simulink model "simulering_ROV_DP_model2"  (R2020a)
settings: Solver=VariableStepAuto  StartTime=0.0  StopTime=t_sim  RelTol=1e-3
values from neighbouring files (symbols this model uses):
  B_aug = [b11 b12 b13 b14 b15 b16 ... (first row only)    [constants.m]
  B_psinv_aug = B_aug'/(B_aug*B_aug')    [constants.m]
  coriolis_effect = 1    [run_simulation.m]    (also in run_simulation_STA_controller.m; run_simulation_dp_model.m)
  d_11 = 250    [constants.m]    (also in constants_dp_model.m; constants_model_coriolis.m; constants_process_model.m)
  d_22 = 200    [constants.m]    (also in constants_dp_model.m; constants_model_coriolis.m; constants_process_model.m)
  d_33 = 175    [constants.m]    (also in constants_dp_model.m; constants_model_coriolis.m; constants_process_model.m)
  d_66 = 15    [constants.m]    (also in constants_process_model.m)
  d_n11 = 350    [constants.m]
  d_n22 = 350    [constants.m]
  d_n33 = 400    [constants.m]
  d_n66 = 75    [constants.m]
  Delta = 25    [plot_simulation_feedback.m]    (also in run_simulation.m; run_simulation_SM_controller.m; run_simulation_STA_controller.m; run_simulation_dp_model.m)
  g_z = 9.81    [run_simulation_FL_controller.m]    (also in run_simulation_PID_controller.m = 0.91; run_simulation_SM_controller.m = 0.91; run_simulation_STA_controller.m = 0.91; run_simulation_dp_model.m = 0.91)
  gamma1 = 50    [run_simulation_dp_model.m]    (also in tuning_dp_model.m = 5)
  gamma2 = 35    [run_simulation_dp_model.m]    (also in tuning_dp_model.m = 3.5)
  gamma_e1 = 0.05    [tuning_dp_model.m]
  gamma_e2 = 0.05    [tuning_dp_model.m]
  gamma_e3 = 0.05    [tuning_dp_model.m]
  k_d_psi = 2*m_44*zeta_d_psi*wn_psi-d_44    [run_simulation_PID_controller.m]    (also in run_simulation_SM_controller.m = 10; run_simulation_dp_model.m = 2*m_66*zeta_d_psi*wn_psi-d_66; run_simulation_feedback_linearizing.m = (2*1*k_p_psi*1-d33/(m_A33+m_RB33)); tuning_PID_controller.m = 2*m_66*zeta_d_psi*wn_psi-d_66)
  k_d_z = 30    [run_simulation_SM_controller.m]    (also in run_simulation_dp_model.m = 2*m_33*zeta_d_heave*wn_heave-d_33; tuning_FL_controller.m = 2*m_33*zeta_d_heave*wn_heave-d_33; tuning_SM_controller.m; tuning_dp_model.m = 2*m_33*zeta_d_heave*wn_heave-d_33)
  k_i_z = wn_heave/10*k_p_z    [run_simulation_PID_controller.m]    (also in run_simulation_dp_model.m = wn_heave/50*k_p_z; tuning_FL_controller.m = wn_heave/50*k_p_z; tuning_PID_controller.m = wn_heave/50*k_p_z; tuning_dp_model.m = wn_heave/50*k_p_z)
  k_p_psi = wn_psi^2-lambda*k_p_r    [run_simulation_FL_controller.m]    (also in run_simulation_PID_controller.m = wn_psi^2*m_44; run_simulation_dp_model.m = wn_psi^2*m_66; run_simulation_feedback_linearizing.m = tau_r_max/deg2rad(45); run_simulation_feedback_linearizing_second_try.m = wn_psi^2*m_44)
  k_p_u = m_11*pole_u-d_11    [run_simulation_FL_controller.m]    (also in run_simulation_PID_controller.m = 10; run_simulation_dp_model.m = pole_u-d_11/m_11; run_simulation_feedback_linearizing.m = tau_u_max/100; run_simulation_feedback_linearizing_second_try.m = 1)
  k_p_v = m_22*pole_v-d_22    [run_simulation_FL_controller.m]    (also in run_simulation_PID_controller.m = 10; run_simulation_dp_model.m = pole_v-d_22/m_22; run_simulation_feedback_linearizing.m = tau_v_max/100; run_simulation_feedback_linearizing_second_try.m = 1)
  k_p_z = wn_heave^2*m_33    [run_simulation_PID_controller.m]    (also in run_simulation_dp_model.m; tuning_FL_controller.m; tuning_PID_controller.m; tuning_dp_model.m)
  m_11 = m_RB11+m_A11    (= 144)    [constants.m]    (also in constants_dp_model.m; constants_model_coriolis.m; constants_process_model.m)
  m_22 = m_RB22+m_A22    (= 162)    [constants.m]    (also in constants_dp_model.m; constants_model_coriolis.m; constants_process_model.m)
  m_66 = m_RB66+m_A66    (= 18.2)    [constants.m]    (also in constants_process_model.m)
  m_A11 = 54    [constants.m]    (also in constants_dp_model.m; constants_model_coriolis.m; constants_process_model.m)
  m_A22 = 72    [constants.m]    (also in constants_dp_model.m; constants_model_coriolis.m; constants_process_model.m)
  m_A33 = 360    [constants.m]    (also in constants_dp_model.m; constants_model_coriolis.m; constants_process_model.m)
  m_A66 = 5.2    [constants.m]    (also in constants_process_model.m)
  m_RB11 = 90    [constants.m]    (also in constants_dp_model.m; constants_model_coriolis.m; constants_process_model.m)
  m_RB22 = 90    [constants.m]    (also in constants_dp_model.m; constants_model_coriolis.m; constants_process_model.m)
  m_RB33 = 90    [constants.m]    (also in constants_dp_model.m; constants_model_coriolis.m; constants_process_model.m)
  m_RB66 = 13    [constants.m]    (also in constants_process_model.m)
  N_nodes = N_elements +1    (= 1001)    [plot_simulation_dp.m]    (also in plot_simulation_feedback.m)
  nonlinear_damping = 0    [run_simulation.m]    (also in run_simulation_STA_controller.m = 1; run_simulation_dp_model.m = 1)
  omega_ref = 1.5    [run_simulation.m]    (also in run_simulation_FL_controller.m = 0.4; run_simulation_PID_controller.m = 0.4; run_simulation_SM_controller.m; run_simulation_STA_controller.m)
  psi0 = deg2rad(psi0)    [constants.m]    (also in constants_dp_model.m; constants_model_coriolis.m; constants_process_model.m)
  psi_r = deg2rad(-45)    [run_simulation.m]    (also in run_simulation_SM_controller.m; run_simulation_STA_controller.m; run_simulation_dp_model.m)
  psi_r1 = deg2rad(psi_r1)    [run_simulation.m]    (also in run_simulation_FL_controller.m = 45; run_simulation_PID_controller.m = 45; run_simulation_SM_controller.m; run_simulation_STA_controller.m)
  psi_r2 = deg2rad(psi_r2)    [run_simulation.m]    (also in run_simulation_FL_controller.m = 90; run_simulation_PID_controller.m = 90; run_simulation_SM_controller.m; run_simulation_STA_controller.m)
  r0 = 0    [constants.m]    (also in constants_dp_model.m; constants_model_coriolis.m; constants_process_model.m)
  step_response = 1    [plot_simulation_feedback.m]    (also in run_simulation.m; run_simulation_SM_controller.m; run_simulation_STA_controller.m; run_simulation_dp_model.m)
  T_ref = 0.2    [run_simulation.m]    (also in run_simulation_FL_controller.m; run_simulation_PID_controller.m; run_simulation_SM_controller.m; run_simulation_STA_controller.m)
  tau_r_max = sqrt(torque_co'*torque_co)    [constants.m]    (also in constants_dp_model.m; constants_model_coriolis.m; constants_process_model.m; run_simulation_feedback_linearizing.m = sqrt(torque_co'*torque_co)/(m_A33+m_RB33))
  tau_u_max = (F_max*cos(alpha1)+F_max*cos(alpha2)+F_max*cos(alpha3)+F_max*cos(alpha4))    [constants.m]    (also in constants_dp_model.m; constants_model_coriolis.m; constants_process_model.m; run_simulation_feedback_linearizing.m = (F_max*cos(alpha1)+F_max*cos(alpha2)+F_max*cos(alpha3)+F_max)
  tau_v_max = (F_max*sin(alpha1)-F_max*sin(alpha2)+F_max*sin(alpha3)-F_max*sin(alpha4))    [constants.m]    (also in constants_dp_model.m; constants_model_coriolis.m; constants_process_model.m; run_simulation_feedback_linearizing.m = (F_max*sin(alpha1)-F_max*sin(alpha2)+F_max*sin(alpha3)-F_max)
  tau_w_max = 2*F_max    (= 240)    [constants.m]    (also in constants_dp_model.m; constants_model_coriolis.m; constants_process_model.m)
  time_step = 700    [run_simulation.m]    (also in run_simulation_SM_controller.m; run_simulation_STA_controller.m; run_simulation_dp_model.m)
  u0 = 0    [constants.m]    (also in constants_dp_model.m; constants_model_coriolis.m; constants_process_model.m)
  u_r = 0.14    [run_simulation.m]    (also in run_simulation_FL_controller.m = 0.2; run_simulation_PID_controller.m = 0.2; run_simulation_SM_controller.m; run_simulation_STA_controller.m)
  v0 = 0    [constants.m]    (also in constants_dp_model.m; constants_model_coriolis.m; constants_process_model.m)
  v_r = 0.14    [run_simulation.m]    (also in run_simulation_FL_controller.m = 0; run_simulation_PID_controller.m = 0; run_simulation_SM_controller.m; run_simulation_STA_controller.m)
  w0 = 0    [constants.m]    (also in constants_dp_model.m; constants_model_coriolis.m; constants_process_model.m)
  x0 = -2*50    (= -100)    [constants.m]    (also in constants_dp_model.m = 0; constants_model_coriolis.m = 0; constants_process_model.m = 0)
  y0 = 0    [constants.m]    (also in constants_dp_model.m; constants_model_coriolis.m; constants_process_model.m)
  z0 = 0    [constants.m]    (also in constants_dp_model.m; constants_model_coriolis.m; constants_process_model.m)
  z_r = 10    [run_simulation.m]    (also in run_simulation_FL_controller.m = 1; run_simulation_PID_controller.m = 1; run_simulation_SM_controller.m; run_simulation_STA_controller.m)
  zeta_ref = 1    [run_simulation.m]    (also in run_simulation_FL_controller.m; run_simulation_PID_controller.m; run_simulation_SM_controller.m; run_simulation_STA_controller.m)
undefined symbols (not defined in the file or in its folder): alpha_k, radius_lim, waypoints
(part 2 of 2)

== system simulering_ROV_DP_model2/Process plant model/Kinetics/Nonlinear damping u ==
  u : Inport
  V_x : Inport  Port=2
  V_y : Inport  Port=3
  psi : Inport  Port=4
  Abs : Abs
  Cos : Trigonometry  Operator=cos
  Gain : Gain  Gain=d_n11
  Product : Product
  Product4 : Product
  Product5 : Product
  Sin : Trigonometry
  Sum : Sum  Inputs=++|
  Sum1 : Sum  Inputs=-+|
  To Workspace : ToWorkspace  VariableName=u_relative_vel  SaveFormat=Structure With Time  SampleTime=-1
  D_n(nu_r)nu_r(1) : Outport
  wires:
  Gain/1 -> Product/1
  Product/1 -> D_n(nu_r)nu_r(1)/1
  Abs/1 -> Gain/1
  psi/1 -> Sin/1, Cos/1
  Sin/1 -> [sinpsi]
  Cos/1 -> [cospsi]
  [V_y] -> Product5/2
  [sinpsi] -> Product5/1
  Product4/1 -> Sum/2
  [V_x] -> Product4/2
  [cospsi] -> Product4/1
  Product5/1 -> Sum/1
  V_x/1 -> [V_x]
  V_y/1 -> [V_y]
  u/1 -> Sum1/2
  Sum1/1 -> To Workspace/1, Product/2, Abs/1
  Sum/1 -> Sum1/1

== system simulering_ROV_DP_model2/Process plant model/Kinetics/Nonlinear damping v ==
  v : Inport
  V_x : Inport  Port=2
  V_y : Inport  Port=3
  psi : Inport  Port=4
  Abs : Abs
  Cos : Trigonometry  Operator=cos
  Gain : Gain  Gain=d_n22
  Product : Product
  Product4 : Product
  Product5 : Product
  Sin : Trigonometry
  Sum : Sum  Inputs=+-|
  Sum1 : Sum  Inputs=-+|
  To Workspace : ToWorkspace  VariableName=v_relative_vel  SaveFormat=Structure With Time  SampleTime=-1
  D_n(nu_r)nu_r(2) : Outport
  wires:
  Gain/1 -> Product/1
  Product/1 -> D_n(nu_r)nu_r(2)/1
  Abs/1 -> Gain/1
  psi/1 -> Sin/1, Cos/1
  Sin/1 -> [sinpsi]
  Cos/1 -> [cospsi]
  [V_y] -> Product5/2
  Product4/1 -> Sum/2
  [V_x] -> Product4/2
  Product5/1 -> Sum/1
  V_x/1 -> [V_x]
  V_y/1 -> [V_y]
  v/1 -> Sum1/2
  Sum1/1 -> To Workspace/1, Product/2, Abs/1
  Sum/1 -> Sum1/1
  [sinpsi] -> Product4/1
  [cospsi] -> Product5/1

== system simulering_ROV_DP_model2/Process plant model/Kinetics/Nonlinear damping w ==
  w : Inport
  Abs : Abs
  Gain : Gain  Gain=d_n33
  Product : Product
  D_n(nu_r)nu_r(3) : Outport
  wires:
  Abs/1 -> Gain/1
  Product/1 -> D_n(nu_r)nu_r(3)/1
  Gain/1 -> Product/1
  w/1 -> Abs/1, Product/2
